simulink model "ex"  (R2025a)
settings: Solver=VariableStepAuto  StartTime=0.0  StopTime=50  RelTol=1e-3
settings Model: Creator=sphuwaset_ros  LastModifiedBy=sphuwaset_ros

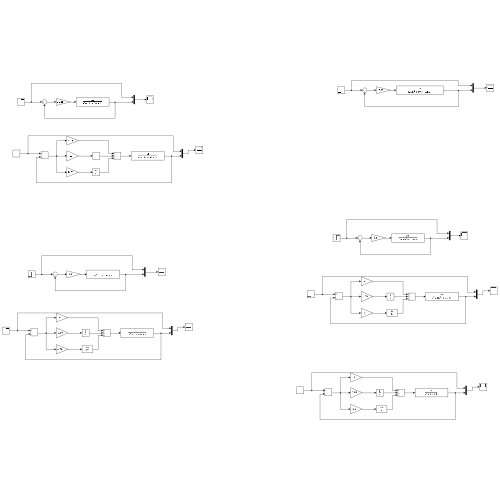
[thumbnail: Simulink's stored preview of the top-level diagram]
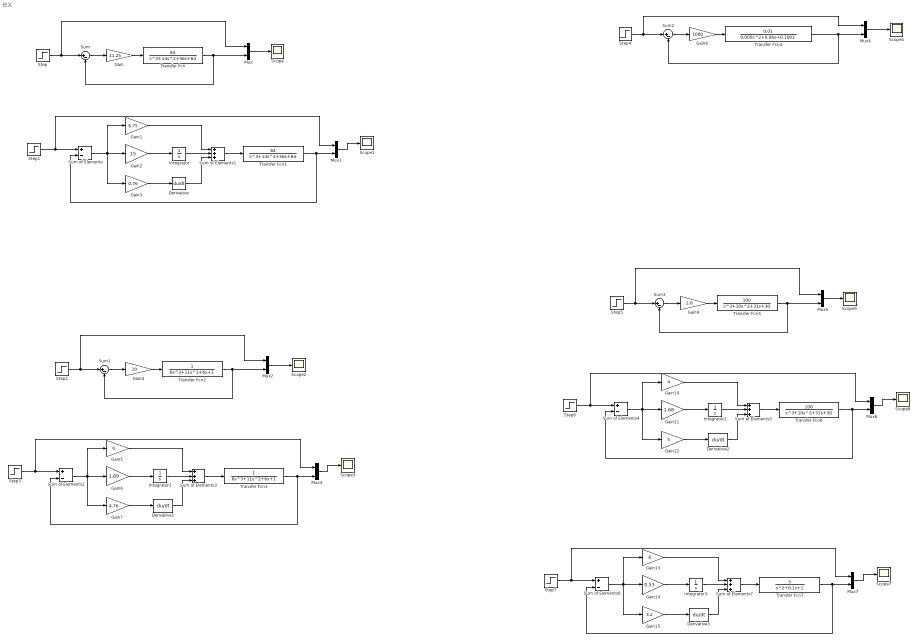
== system ex ==
  Derivative{,1..3} (4 alike) : Derivative
  Gain : Gain  Gain=11.25
  Gain1 : Gain  Gain=6.75
  Gain10 : Gain  Gain=4
  Gain11 : Gain  Gain=1.68
  Gain12 : Gain  Gain=5
  Gain13 : Gain  Gain=8
  Gain14 : Gain  Gain=0.53
  Gain15 : Gain  Gain=3.2
  Gain2 : Gain  Gain=15
  Gain3 : Gain  Gain=0.76
  Gain4 : Gain  Gain=10
  Gain5 : Gain  Gain=6
  Gain6 : Gain  Gain=1.89
  Gain7 : Gain  Gain=4.76
  Gain8 : Gain  Gain=1000
  Gain9 : Gain  Gain=2.8
  Integrator{,1..3} (4 alike) : Integrator
  Mux{,1..7} (8 alike) : Mux  Inputs=2
  Scope{,1..7} (8 alike) : Scope
      Scope settings: ActiveDisplayYMinimum=-0.47684951882591919  ActiveDisplayYMaximum=2.1835372913212852
      Scope1 settings: ActiveDisplayYMinimum=-0.378316477727213  ActiveDisplayYMaximum=2.6079645253271426
      Scope2 settings: ActiveDisplayYMinimum=-0.59024759040087127  ActiveDisplayYMaximum=3.74324218979749  DataLoggingVariableName=ScopeData2
      Scope3 settings: ActiveDisplayYMinimum=-0.24653019425452416  ActiveDisplayYMaximum=1.7342641346564955  DataLoggingVariableName=ScopeData3
      Scope4 settings: ActiveDisplayYMinimum=0.80331688379608757  ActiveDisplayYMaximum=1.1543632504809931  DataLoggingVariableName=ScopeData4
      Scope5 settings: ActiveDisplayYMinimum=0.13876946859217254  ActiveDisplayYMaximum=2.3909333730333491  DataLoggingVariableName=ScopeData5
      Scope6 settings: ActiveDisplayYMinimum=-0.2485743338381069  ActiveDisplayYMaximum=1.8286192259238268  DataLoggingVariableName=ScopeData6
      Scope7 settings: ActiveDisplayYMinimum=-0.2485743338381069  ActiveDisplayYMaximum=1.8286192259238268  DataLoggingVariableName=ScopeData7
  Step{,2,4..5} (4 alike) : Step  Time=0  SampleTime=0  ZeroCross=off
  Step1 : Step  SampleTime=0
  Step3 : Step  SampleTime=0
  Step6 : Step  Time=0  SampleTime=0
  Step7 : Step  Time=0  SampleTime=0
  Sum{,1..3} (4 alike) : Sum  Inputs=|+-
  Sum of Elements{,2,4,6} (4 alike) : Sum  Inputs=+-
  Sum of Elements{1,3,5,7} (4 alike) : Sum  Inputs=+++
  Transfer Fcn : TransferFcn  Numerator=[64]  Denominator=[1 14 56 64]
  Transfer Fcn1 : TransferFcn  Numerator=[64]  Denominator=[1 14 56 64]
  Transfer Fcn2 : TransferFcn  Denominator=[6 11 6 1]
  Transfer Fcn3 : TransferFcn  Denominator=[6 11 6 1]
  Transfer Fcn4 : TransferFcn  Numerator=[0.01]  Denominator=[0.005 0.06 0.1001]
  Transfer Fcn5 : TransferFcn  Numerator=[100]  Denominator=[1 10 31 30]
  Transfer Fcn6 : TransferFcn  Numerator=[100]  Denominator=[1 10 31 30]
  Transfer Fcn7 : TransferFcn  Numerator=[5]  Denominator=[1 0.1 1]
  wires:
  Gain/1 -> Transfer Fcn/1
  Transfer Fcn/1 -> Sum/2, Mux/2
  Sum/1 -> Gain/1
  Step/1 -> Sum/1, Mux/1
  Mux/1 -> Scope/1
  Step1/1 -> Mux1/1, Sum of Elements/1
  Sum of Elements/1 -> Gain3/1, Gain1/1, Gain2/1
  Gain2/1 -> Integrator/1
  Gain1/1 -> Sum of Elements1/1
  Integrator/1 -> Sum of Elements1/2
  Gain3/1 -> Derivative/1
  Derivative/1 -> Sum of Elements1/3
  Sum of Elements1/1 -> Transfer Fcn1/1
  Transfer Fcn1/1 -> Mux1/2, Sum of Elements/2
  Mux1/1 -> Scope1/1
  Mux2/1 -> Scope2/1
  Transfer Fcn2/1 -> Sum1/2, Mux2/2
  Sum1/1 -> Gain4/1
  Step2/1 -> Sum1/1, Mux2/1
  Gain4/1 -> Transfer Fcn2/1
  Gain6/1 -> Integrator1/1
  Sum of Elements2/1 -> Gain7/1, Gain5/1, Gain6/1
  Step3/1 -> Mux3/1, Sum of Elements2/1
  Gain7/1 -> Derivative1/1
  Mux3/1 -> Scope3/1
  Transfer Fcn3/1 -> Mux3/2, Sum of Elements2/2
  Sum of Elements3/1 -> Transfer Fcn3/1
  Gain5/1 -> Sum of Elements3/1
  Integrator1/1 -> Sum of Elements3/2
  Derivative1/1 -> Sum of Elements3/3
  Step4/1 -> Sum2/1, Mux4/1
  Sum2/1 -> Gain8/1
  Transfer Fcn4/1 -> Sum2/2, Mux4/2
  Gain8/1 -> Transfer Fcn4/1
  Mux4/1 -> Scope4/1
  Transfer Fcn5/1 -> Sum3/2, Mux5/2
  Step6/1 -> Mux6/1, Sum of Elements4/1
  Transfer Fcn6/1 -> Mux6/2, Sum of Elements4/2
  Mux6/1 -> Scope6/1
  Derivative2/1 -> Sum of Elements5/3
  Gain10/1 -> Sum of Elements5/1
  Gain9/1 -> Transfer Fcn5/1
  Sum of Elements4/1 -> Gain12/1, Gain10/1, Gain11/1
  Step5/1 -> Sum3/1, Mux5/1
  Sum of Elements5/1 -> Transfer Fcn6/1
  Gain11/1 -> Integrator2/1
  Integrator2/1 -> Sum of Elements5/2
  Mux5/1 -> Scope5/1
  Gain12/1 -> Derivative2/1
  Sum3/1 -> Gain9/1
  Gain14/1 -> Integrator3/1
  Derivative3/1 -> Sum of Elements7/3
  Mux7/1 -> Scope7/1
  Transfer Fcn7/1 -> Mux7/2, Sum of Elements6/2
  Integrator3/1 -> Sum of Elements7/2
  Sum of Elements6/1 -> Gain15/1, Gain13/1, Gain14/1
  Gain15/1 -> Derivative3/1
  Step7/1 -> Mux7/1, Sum of Elements6/1
  Gain13/1 -> Sum of Elements7/1
  Sum of Elements7/1 -> Transfer Fcn7/1
